simulink model "DVBS2BentPipeLinkModel"  (R2021b)
settings: Solver=VariableStepAuto  StartTime=0.0  StopTime=0.025  RelTol=1e-3
PreLoadFcn:
  | modulationAndCodingMode = 'QPSK 1/4';
  | seed = 25;
  | ldpcFrameLength = 'Normal';
  | selDPD = false;
  | ulFreq = 4;  % GHz
  | selLvlBO = 1;  % '30 dB  (negligible nonlinearity)'
  | gsTxAntDiam = 4;  % m
  | selDoppler = 1;  %'0 Hz'
  | filterSpanInSymbols = 6;
  | sampPerSym = 8;
  | altitude = 35600;  % km
  | satRxAntDiam = 0.3;  % m
  | satRxNoiseFigure = 6;  % dB
  | chebyFilterOrder = 4;
  | satHPABackoff = 8;  % dB
  | dlFreq = 4.2;  % GHz
  | satTxAntDiam = 0.3;  % m
  | gsRxAntDiam = 1;  % m
  | gsRxNoiseFigure = 3;  % dB
  | selPhNo = 1;  % 'Negligible (-100 dBc/Hz @ 100 Hz)'
  | iqAmpImbal = 0;  % dB
  | iqPhImbal = 0;  % deg
  | dcOffsetPct = 0;  % percent of mean in-phase voltage
  | selDcOffset = false;
  | selCorrIQ = false;
  | selCorrDoppler = false;
  | LDPCNumIterations = 50;
  | DVBS2BentPipeInit(modulationAndCodingMode, seed, ...
  |   ldpcFrameLength, selDPD, ...
  |   ulFreq, selLvlBO, gsTxAntDiam, selDoppler, ...
  |   filterSpanInSymbols, sampPerSym, ...
  |   altitude, satRxAntDiam, satRxNoiseFigure, ...
  |   chebyFilterOrder, satHPABackoff, dlFreq, satTxAntDiam, ...
  |   gsRxAntDiam, gsRxNoiseFigure, selPhNo, ...
  |   iqAmpImbal, iqPhImbal, dcOffsetPct, ...
  |   selDcOffset, selCorrIQ, selCorrDoppler, ...
  |   LDPCNumIterations);
  | 
  | clear modulationAndCodingMode seed ldpcFrameLength selDPD
  | clear ulFreq selLvlBO gsTxAntDiam selDoppler
  | clear filterSpanInSymbols sampPerSym
  | clear altitude satRxAntDiam satRxNoiseFigure
  | clear chebyFilterOrder satHPABackoff dlFreq satTxAntDiam
  | clear gsRxAntDiam gsRxNoiseFigure selPhNo
  | clear iqAmpImbal iqPhImbal dcOffsetPct
  | clear selDcOffset selCorrIQ selCorrDoppler
  | clear LDPCNumIterations
undefined symbols (not defined in the file or in its folder): paramRFSatLink
libraries: dspstat3 x17, commrflib2 x9, commrfcorlib x5, commblkcod2 x4, dspsigops x4, commsink2 x3, commutil2 x3, dspmathops x3, commblkintrlv2 x2, dspobslib x2, commdigbbndpm3 x2, commfilt2 x2
(part 2 of 2)

== matlab function DVBS2BentPipeLinkModel/Estimate Noise Variance/Estimate Noise Variance ==
  data: x input; estVar output; modIdx input
function estVar = estimateNoiseVariance(x,modIdx)
% ESTIMATENOISEVARIANCE Estimate noise variance of an input signal
%
% ESTVAR = ESTIMATENOISEVARIANCE(X,MODTYPE) returns the estimated noise
% variance in a noisy signal X with modulation type MODTYPE.  X is a
% complex scalar or column vector, and MODIDX is either 1, for QPSK, or 2,
% for 8PSK.

if modIdx == 1  % QPSK
  refSig = repmat([0.707106781186548 + 0.707106781186547i ...
                  -0.707106781186547 + 0.707106781186548i ...
                  -0.707106781186548 - 0.707106781186547i ...
                   0.707106781186547 - 0.707106781186548i], ...
                   length(x),1);
else  % 8PSK
  refSig = repmat([0.923879532511287 + 0.382683432365090i ...
                   0.382683432365090 + 0.923879532511287i ...
                  -0.382683432365090 + 0.923879532511287i ...
                  -0.923879532511287 + 0.382683432365090i ...
                  -0.923879532511287 - 0.382683432365090i ...
                  -0.382683432365090 - 0.923879532511287i ...
                   0.382683432365090 - 0.923879532511287i ...
                   0.923879532511287 - 0.382683432365090i], ...
                   length(x),1);
end

x = repmat(x,1,size(refSig,2));
tmp1 = x - refSig;
dist = real(tmp1).^2 + imag(tmp1).^2; % all possible constellation points
[~,colIdx] = min(dist,[],2);
rowIdx = (1:length(x))';
idx = sub2ind(size(dist),rowIdx,colIdx);  % linear indexing
noise = tmp1(idx);
estVar = var(noise);
